simulink model "Test_Word_Multiplexer_8_to_1"  (R2023a)
settings: Solver=ode45  StartTime=0.0  StopTime=len  RelTol=1e-3  EnableMultiTasking=on
libraries: Miscellaneous x9, simulink x1, Word_Multiplexers_Lib x1
settings Model: Creator=N  LastModifiedBy=Jozko Mrkvicka
settings SolverCC: AlgebraicLoopSolver=TrustRegion
settings DataIOCC: SaveFormat=Array  ReturnWorkspaceOutputs=off
settings OptimizationCC: LifeSpan=inf
settings DebuggingCC: UnconnectedInputMsg=warning  UnconnectedOutputMsg=warning  UnconnectedLineMsg=warning  SFUnexpectedBacktrackingDiag=warning  SFNoUnconditionalDefaultTransitionDiag=warning  ArithmeticOperatorsInVariantConditions=warning
settings HardwareCC: ProdWordSize=32
settings ModelReferenceCC: EnableRefExpFcnMdlSchedulingChecks=on
settings SFSimCC: SimUseLocalCustomCode=off  CustomCodeUndefinedFunction=UseInterfaceOnly
settings RTWCC: RTWUseLocalCustomCode=off
settings CodeAppCC: StateflowObjectComments=on
settings GRTTargetCC: TargetLangStandard=C89/C90 (ANSI)
settings ConfigComp: CovMetricSettings=dw  CovSaveCumulativeToWorkspaceVar=on  CovSaveSingleToWorkspaceVar=on  CovExternalEMLEnable=off

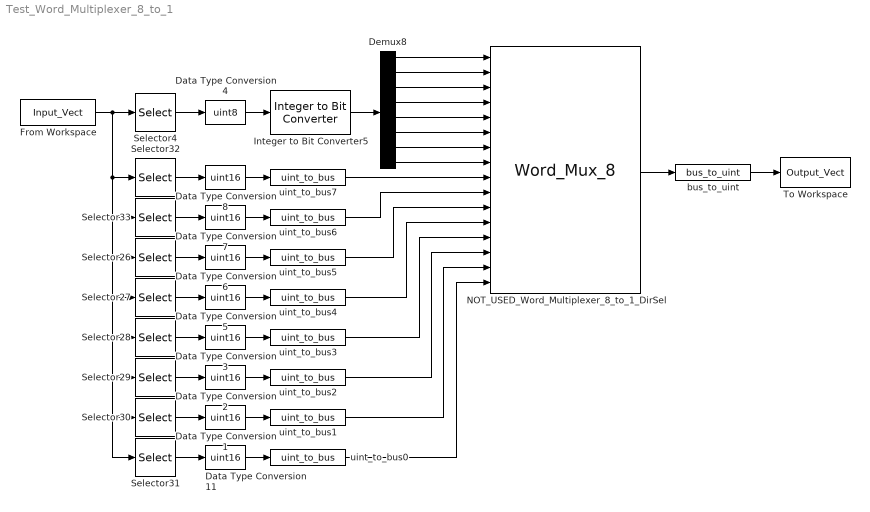
== system Test_Word_Multiplexer_8_to_1 ==
  Data Type Conversion{1..3,5..8,11} (8 alike) : DataTypeConversion  OutDataTypeStr=uint16  SaturateOnIntegerOverflow=off  RndMeth=Floor
  Data Type Conversion4 : DataTypeConversion  OutDataTypeStr=uint8  SaturateOnIntegerOverflow=off  RndMeth=Floor
  Demux8 : Demux  Outputs=8
  From Workspace : FromWorkspace  VariableName=Input_Vect  SampleTime=1  Interpolate=off  ZeroCross=off  OutputAfterFinalValue=Holding final value
  Integer to Bit Converter5 : simulink/Logic and Bit Operations/Integer to Bit Converter  nbits=8  signedInputValues=Unsigned  bitOrder=MSB first  outDtype=boolean
      settings: LibrarySourceBlock=|
      | commutil2/Integer to Bit
      | Converter
  NOT_USED_Word_Multiplexer_8_to_1_DirSel : Word_Multiplexers_Lib/Word_Mux_8  SystemSampleTime=-1  VariantActivationTime=update diagram  Latency=0  AutoFrameSizeCalculation=off
  Selector26 : Selector  IndexMode=Zero-based  InputPortWidth=9  IndexOptions=Index vector (dialog)  Indices=3  OutputSizes=1
  Selector27 : Selector  IndexMode=Zero-based  InputPortWidth=9  IndexOptions=Index vector (dialog)  Indices=4  OutputSizes=1
  Selector28 : Selector  IndexMode=Zero-based  InputPortWidth=9  IndexOptions=Index vector (dialog)  Indices=5  OutputSizes=1
  Selector29 : Selector  IndexMode=Zero-based  InputPortWidth=9  IndexOptions=Index vector (dialog)  Indices=6  OutputSizes=1
  Selector30 : Selector  IndexMode=Zero-based  InputPortWidth=9  IndexOptions=Index vector (dialog)  Indices=7  OutputSizes=1
  Selector31 : Selector  IndexMode=Zero-based  InputPortWidth=9  IndexOptions=Index vector (dialog)  Indices=8  OutputSizes=1
  Selector32 : Selector  IndexMode=Zero-based  InputPortWidth=9  IndexOptions=Index vector (dialog)  Indices=1  OutputSizes=1
  Selector33 : Selector  IndexMode=Zero-based  InputPortWidth=9  IndexOptions=Index vector (dialog)  Indices=2  OutputSizes=1
  Selector4 : Selector  IndexMode=Zero-based  InputPortWidth=9  SampleTime=1  IndexOptions=Index vector (dialog)  Indices=0  OutputSizes=1
  To Workspace : ToWorkspace  VariableName=Output_Vect  SampleTime=1
  bus_to_uint : Miscellaneous/bus_to_uint  SystemSampleTime=-1  VariantActivationTime=update diagram  Latency=0  AutoFrameSizeCalculation=off
  uint_to_bus{0..7} (8 alike) : Miscellaneous/uint_to_bus  SystemSampleTime=-1  VariantActivationTime=update diagram  Latency=0  AutoFrameSizeCalculation=off
  wires:
  Integer to Bit Converter5/1 -> Demux8/1
  NOT_USED_Word_Multiplexer_8_to_1_DirSel/1 -> bus_to_uint/1
  Selector4/1 -> Data Type Conversion4/1
  Data Type Conversion4/1 -> Integer to Bit Converter5/1
  From Workspace/1 -> Selector4/1, Selector32/1, Selector33/1, Selector26/1, Selector27/1, Selector28/1, Selector29/1, Selector30/1, Selector31/1
  Selector32/1 -> Data Type Conversion8/1
  Selector33/1 -> Data Type Conversion7/1
  Selector26/1 -> Data Type Conversion6/1
  Selector27/1 -> Data Type Conversion5/1
  Selector28/1 -> Data Type Conversion3/1
  Selector29/1 -> Data Type Conversion2/1
  Selector30/1 -> Data Type Conversion1/1
  Selector31/1 -> Data Type Conversion11/1
  Data Type Conversion8/1 -> uint_to_bus7/1
  Data Type Conversion7/1 -> uint_to_bus6/1
  Data Type Conversion6/1 -> uint_to_bus5/1
  Data Type Conversion5/1 -> uint_to_bus4/1
  Data Type Conversion3/1 -> uint_to_bus3/1
  Data Type Conversion2/1 -> uint_to_bus2/1
  Data Type Conversion1/1 -> uint_to_bus1/1
  Data Type Conversion11/1 -> uint_to_bus0/1
  bus_to_uint/1 -> To Workspace/1
  uint_to_bus0/1 -> NOT_USED_Word_Multiplexer_8_to_1_DirSel/16
  uint_to_bus1/1 -> NOT_USED_Word_Multiplexer_8_to_1_DirSel/15
  uint_to_bus2/1 -> NOT_USED_Word_Multiplexer_8_to_1_DirSel/14
  uint_to_bus3/1 -> NOT_USED_Word_Multiplexer_8_to_1_DirSel/13
  uint_to_bus4/1 -> NOT_USED_Word_Multiplexer_8_to_1_DirSel/12
  uint_to_bus5/1 -> NOT_USED_Word_Multiplexer_8_to_1_DirSel/11
  uint_to_bus6/1 -> NOT_USED_Word_Multiplexer_8_to_1_DirSel/10
  uint_to_bus7/1 -> NOT_USED_Word_Multiplexer_8_to_1_DirSel/9
  Demux8/1 -> NOT_USED_Word_Multiplexer_8_to_1_DirSel/1
  Demux8/2 -> NOT_USED_Word_Multiplexer_8_to_1_DirSel/2
  Demux8/3 -> NOT_USED_Word_Multiplexer_8_to_1_DirSel/3
  Demux8/4 -> NOT_USED_Word_Multiplexer_8_to_1_DirSel/4
  Demux8/5 -> NOT_USED_Word_Multiplexer_8_to_1_DirSel/5
  Demux8/6 -> NOT_USED_Word_Multiplexer_8_to_1_DirSel/6
  Demux8/7 -> NOT_USED_Word_Multiplexer_8_to_1_DirSel/7
  Demux8/8 -> NOT_USED_Word_Multiplexer_8_to_1_DirSel/8
